simulink model "UpgradedConveyorBeltMechanism"  (R2023a)
settings: Solver=VariableStepAuto  StartTime=0.0  StopTime=30  RelTol=1e-3
values from neighbouring files (symbols this model uses):
  b = 40.6518    [UpgradedConveyorBeltParameters.m]
  B1 = 0.0042    [UpgradedConveyorBeltParameters.m]
  B2 = 0.0084    [UpgradedConveyorBeltParameters.m]
  J1 = 7e-5    (= 7e-05)    [UpgradedConveyorBeltParameters.m]
  J2 = 8e-5    (= 8e-05)    [UpgradedConveyorBeltParameters.m]
  k1 = 2.6552e5    (= 265520)    [UpgradedConveyorBeltParameters.m]
  k2 = 2.6552e5    (= 265520)    [UpgradedConveyorBeltParameters.m]
  k3 = 11.777e4    (= 117770)    [UpgradedConveyorBeltParameters.m]
  Kb = 23e-3    (= 0.023)    [UpgradedConveyorBeltParameters.m]
  Kt = 23e-3    (= 0.023)    [UpgradedConveyorBeltParameters.m]
  L = 0.1    [UpgradedConveyorBeltParameters.m]
  m = 2    [UpgradedConveyorBeltParameters.m]
  R = 0.71    [UpgradedConveyorBeltParameters.m]
  r = 0.0194    [UpgradedConveyorBeltParameters.m]
undefined symbols (not defined in the file or in its folder): J, Kd, Ke
libraries: fl_lib x20, slpidlib x10, fl_ps_legacy_lib x8, nesl_utility x6, SignalEditorBlockLib x5, ee_lib x2, simulink x1
(part 2 of 2)

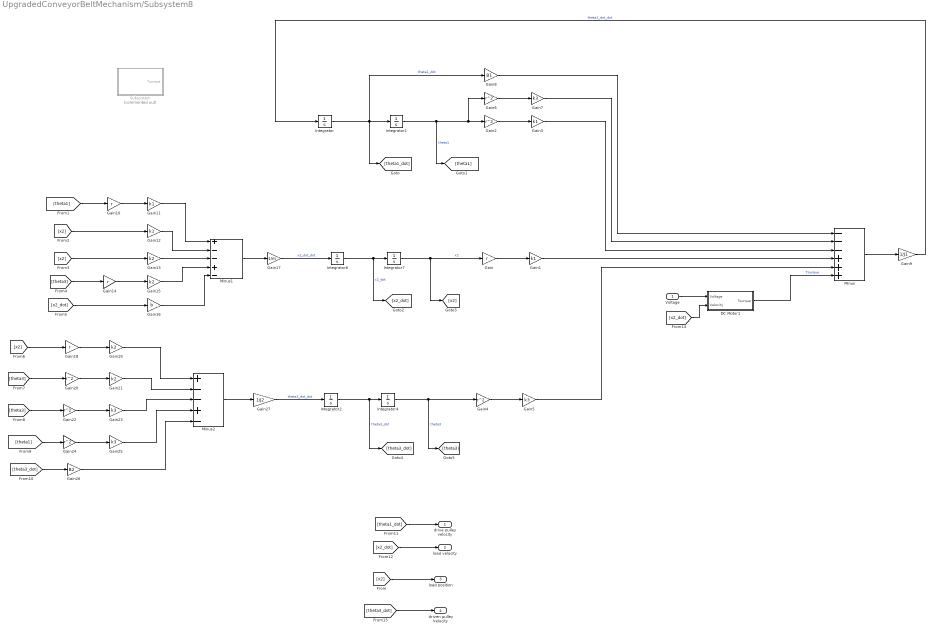
== system UpgradedConveyorBeltMechanism/Subsystem8 ==
  Voltage : Inport
  DC Motor1 : Subsystem
  Gain{,10,14,18} (4 alike) : Gain  Gain=r
  Gain{1,3,11..12} (4 alike) : Gain  Gain=k1
  Gain{13,15,19,21} (4 alike) : Gain  Gain=k2
  Gain16 : Gain  Gain=b
  Gain17 : Gain  Gain=1/m
  Gain{2,4,6,20,22,24} (6 alike) : Gain  Gain=r^2
  Gain{5,7,23,25} (4 alike) : Gain  Gain=k3
  Gain26 : Gain  Gain=B2
  Gain27 : Gain  Gain=1/J2
  Gain8 : Gain  Gain=B1
  Gain9 : Gain  Gain=1/J1
  Integrator{,1..2,4,6..7} (6 alike) : Integrator
  Minus : Sum  Inputs=---+++
  Minus1 : Sum  Inputs=+--+-
  Minus2 : Sum  Inputs=+--+-
  Subsystem : Subsystem  Commented=on
  drive pulley velocity : Outport
  load velocity : Outport  Port=2
  load position : Outport  Port=3
  driven pulley Velocity : Outport  Port=4
  wires:
  Gain23/1 -> Minus2/3
  Gain4/1 -> Gain5/1
  [theta1] -> Gain24/1
  Gain11/1 -> Minus1/1
  [theta3_dot] -> Gain26/1
  Gain26/1 -> Minus2/5
  Gain22/1 -> Gain23/1
  Gain19/1 -> Minus2/1
  Gain21/1 -> Minus2/2
  Integrator/1 -> Integrator1/1, [theta1_dot], Gain8/1  "theta1_dot"
  Integrator1/1 -> Gain6/1, Gain2/1, [theta1]  "theta1"
  Integrator6/1 -> Integrator7/1, [x2_dot]  "x2_dot"
  Gain3/1 -> Minus/3
  Gain18/1 -> Gain19/1
  Gain1/1 -> Minus/4
  Gain2/1 -> Gain3/1
  Integrator2/1 -> [theta3_dot], Integrator4/1  "theta3_dot"
  Integrator4/1 -> Gain4/1, [theta3]  "theta3"
  [x2] -> Gain12/1
  Gain/1 -> Gain1/1
  Gain10/1 -> Gain11/1
  Gain24/1 -> Gain25/1
  Gain13/1 -> Minus1/3
  [theta3] -> Gain20/1
  [theta3] -> Gain14/1
  Gain15/1 -> Minus1/4
  Gain6/1 -> Gain7/1
  [theta3] -> Gain22/1
  Gain5/1 -> Minus/5
  [theta1] -> Gain10/1
  [x2] -> Gain18/1
  Minus2/1 -> Gain27/1
  Minus1/1 -> Gain17/1
  Minus/1 -> Gain9/1
  Gain7/1 -> Minus/2
  Integrator7/1 -> Gain/1, [x2]  "x2"
  Gain16/1 -> Minus1/5
  Gain8/1 -> Minus/1
  Gain17/1 -> Integrator6/1  "x2_dot_dot"
  Gain14/1 -> Gain15/1
  Gain20/1 -> Gain21/1
  Gain9/1 -> Integrator/1  "theta1_dot_dot"
  Gain12/1 -> Minus1/2
  Gain25/1 -> Minus2/4
  [x2] -> Gain13/1
  [x2_dot] -> Gain16/1
  [theta1_dot] -> drive pulley velocity/1
  [x2_dot] -> load velocity/1
  Gain27/1 -> Integrator2/1  "theta3_dot_dot"
  DC Motor1/1(Tourque) -> Minus/6  "Tourque"
  [x2_dot] -> DC Motor1/2(Velocity)
  Voltage/1 -> DC Motor1/1(Voltage)
  [x2] -> load position/1
  [theta3_dot] -> driven pulley Velocity/1

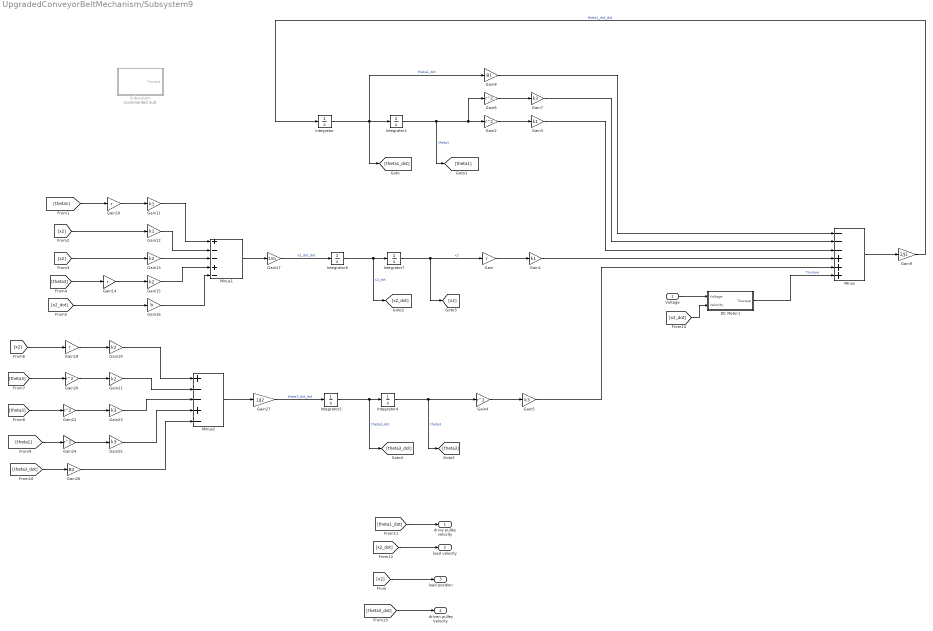
== system UpgradedConveyorBeltMechanism/Subsystem9 ==
  Voltage : Inport
  DC Motor1 : Subsystem
  Gain{,10,14,18} (4 alike) : Gain  Gain=r
  Gain{1,3,11..12} (4 alike) : Gain  Gain=k1
  Gain{13,15,19,21} (4 alike) : Gain  Gain=k2
  Gain16 : Gain  Gain=b
  Gain17 : Gain  Gain=1/m
  Gain{2,4,6,20,22,24} (6 alike) : Gain  Gain=r^2
  Gain{5,7,23,25} (4 alike) : Gain  Gain=k3
  Gain26 : Gain  Gain=B2
  Gain27 : Gain  Gain=1/J2
  Gain8 : Gain  Gain=B1
  Gain9 : Gain  Gain=1/J1
  Integrator{,1..2,4,6..7} (6 alike) : Integrator
  Minus : Sum  Inputs=---+++
  Minus1 : Sum  Inputs=+--+-
  Minus2 : Sum  Inputs=+--+-
  Subsystem : Subsystem  Commented=on
  drive pulley velocity : Outport
  load velocity : Outport  Port=2
  load position : Outport  Port=3
  driven pulley Velocity : Outport  Port=4
  wires:
  Gain23/1 -> Minus2/3
  Gain4/1 -> Gain5/1
  [theta1] -> Gain24/1
  Gain11/1 -> Minus1/1
  [theta3_dot] -> Gain26/1
  Gain26/1 -> Minus2/5
  Gain22/1 -> Gain23/1
  Gain19/1 -> Minus2/1
  Gain21/1 -> Minus2/2
  Integrator/1 -> Integrator1/1, [theta1_dot], Gain8/1  "theta1_dot"
  Integrator1/1 -> Gain6/1, Gain2/1, [theta1]  "theta1"
  Integrator6/1 -> Integrator7/1, [x2_dot]  "x2_dot"
  Gain3/1 -> Minus/3
  Gain18/1 -> Gain19/1
  Gain1/1 -> Minus/4
  Gain2/1 -> Gain3/1
  Integrator2/1 -> [theta3_dot], Integrator4/1  "theta3_dot"
  Integrator4/1 -> Gain4/1, [theta3]  "theta3"
  [x2] -> Gain12/1
  Gain/1 -> Gain1/1
  Gain10/1 -> Gain11/1
  Gain24/1 -> Gain25/1
  Gain13/1 -> Minus1/3
  [theta3] -> Gain20/1
  [theta3] -> Gain14/1
  Gain15/1 -> Minus1/4
  Gain6/1 -> Gain7/1
  [theta3] -> Gain22/1
  Gain5/1 -> Minus/5
  [theta1] -> Gain10/1
  [x2] -> Gain18/1
  Minus2/1 -> Gain27/1
  Minus1/1 -> Gain17/1
  Minus/1 -> Gain9/1
  Gain7/1 -> Minus/2
  Integrator7/1 -> Gain/1, [x2]  "x2"
  Gain16/1 -> Minus1/5
  Gain8/1 -> Minus/1
  Gain17/1 -> Integrator6/1  "x2_dot_dot"
  Gain14/1 -> Gain15/1
  Gain20/1 -> Gain21/1
  Gain9/1 -> Integrator/1  "theta1_dot_dot"
  Gain12/1 -> Minus1/2
  Gain25/1 -> Minus2/4
  [x2] -> Gain13/1
  [x2_dot] -> Gain16/1
  [theta1_dot] -> drive pulley velocity/1
  [x2_dot] -> load velocity/1
  Gain27/1 -> Integrator2/1  "theta3_dot_dot"
  DC Motor1/1(Tourque) -> Minus/6  "Tourque"
  [x2_dot] -> DC Motor1/2(Velocity)
  Voltage/1 -> DC Motor1/1(Voltage)
  [x2] -> load position/1
  [theta3_dot] -> driven pulley Velocity/1

== system UpgradedConveyorBeltMechanism/Controller/Position ==
  Ref : Inport
  Algorithm and Pulse Generation : Subsystem
  ERef : fl_lib/Electrical/Electrical Elements/Electrical Reference
  PWM : PMIOPort  Side=Right
  0v : PMIOPort  Port=2  Side=Right
  REV : PMIOPort  Port=3  Side=Right
  wires:
  Ref/1 -> Algorithm and Pulse Generation/1(Reference)
  connections:
  Algorithm and Pulse Generation/RConn2 -- PWM/RConn1
  Algorithm and Pulse Generation/RConn1 -- REV/RConn1
  ERef/LConn1 -- 0v/RConn1

== system UpgradedConveyorBeltMechanism/Controller/Speed ==
  note: Step rate and direction algorithm implemented on a microprocessor or dedicated discrete chip
  Ref : Inport
  ERef : fl_lib/Electrical/Electrical Elements/Electrical Reference
  Step Rate and Direction : Subsystem
  Voltage-Controlled Pulse Generator : Subsystem
  PWM : PMIOPort  Side=Right
  0v : PMIOPort  Port=2  Side=Right
  REV : PMIOPort  Port=3  Side=Right
  wires:
  Ref/1 -> Step Rate and Direction/1(Reference)
  connections:
  PWM/RConn1 -- Voltage-Controlled Pulse Generator/RConn1
  Voltage-Controlled Pulse Generator/RConn2 -- 0v/RConn1 -- ERef/LConn1
  Step Rate and Direction/RConn1 -- REV/RConn1
  Step Rate and Direction/RConn2 -- Voltage-Controlled Pulse Generator/LConn1

== system UpgradedConveyorBeltMechanism/Subsystem/DC Motor1 ==
  note: Armature Controlled DC Motor
      |
      | $E_a = R_a \cdot I_a + L_a \cdot \frac{di_a}{dt} + K_b \cdot \frac{d\theta}{dt}$
      | $T_{m} = K_{t} \cdot I_{a}$
  Voltage : Inport
  Velocity : Inport  Port=2
  Constant1 : Constant  Value=R
  Gain1 : Gain  Gain=Kb
  Gain2 : Gain  Gain=1/L
  Gain3 : Gain  Gain=Kt
  Integrator : Integrator
  Product : Product
  Subtract : Sum  Inputs=+--
  Tourque : Outport
  wires:
  Voltage/1 -> Subtract/1
  Integrator/1 -> Product/1, Gain3/1  "i"
  Gain3/1 -> Tourque/1
  Gain1/1 -> Subtract/2
  Velocity/1 -> Gain1/1
  Constant1/1 -> Product/2
  Product/1 -> Subtract/3
  Gain2/1 -> Integrator/1  "i_dot"
  Subtract/1 -> Gain2/1

== system UpgradedConveyorBeltMechanism/Subsystem1/DC Motor1 ==
  note: Armature Controlled DC Motor
      |
      | $E_a = R_a \cdot I_a + L_a \cdot \frac{di_a}{dt} + K_b \cdot \frac{d\theta}{dt}$
      | $T_{m} = K_{t} \cdot I_{a}$
  Voltage : Inport
  Velocity : Inport  Port=2
  Constant1 : Constant  Value=R
  Gain1 : Gain  Gain=Kb
  Gain2 : Gain  Gain=1/L
  Gain3 : Gain  Gain=Kt
  Integrator : Integrator
  Product : Product
  Subtract : Sum  Inputs=+--
  Tourque : Outport
  wires:
  Voltage/1 -> Subtract/1
  Integrator/1 -> Product/1, Gain3/1  "i"
  Gain3/1 -> Tourque/1
  Gain1/1 -> Subtract/2
  Velocity/1 -> Gain1/1
  Constant1/1 -> Product/2
  Product/1 -> Subtract/3
  Gain2/1 -> Integrator/1  "i_dot"
  Subtract/1 -> Gain2/1

== system UpgradedConveyorBeltMechanism/Subsystem1/Subsystem ==
  Constant : Constant  Value=Kt
  Constant1 : Constant  Value=Ke
  Constant2 : Constant  Value=R
  Divide : Product  Inputs=**/
  Divide1 : Product  Inputs=***/
  Minus3 : Sum  Inputs=+-
  Voltage : DiscretePulseGenerator  PulseType=Time based  Amplitude=12  Period=11  PulseWidth=50  PhaseDelay=2
  Tourque : Outport
  wires:
  Divide1/1 -> Minus3/2
  Divide/1 -> Minus3/1
  Constant/1 -> Divide/2, Divide1/1
  [theta1_dot] -> Divide1/3
  Constant1/1 -> Divide1/2
  Constant2/1 -> Divide1/4, Divide/3
  Minus3/1 -> Tourque/1  "Tourque"
  Voltage/1 -> Divide/1

== system UpgradedConveyorBeltMechanism/Subsystem10/DC Motor1 ==
  note: Armature Controlled DC Motor
      |
      | $E_a = R_a \cdot I_a + L_a \cdot \frac{di_a}{dt} + K_b \cdot \frac{d\theta}{dt}$
      | $T_{m} = K_{t} \cdot I_{a}$
  Voltage : Inport
  Velocity : Inport  Port=2
  Constant1 : Constant  Value=R
  Gain1 : Gain  Gain=Kb
  Gain2 : Gain  Gain=1/L
  Gain3 : Gain  Gain=Kt
  Integrator : Integrator
  Product : Product
  Subtract : Sum  Inputs=+--
  Tourque : Outport
  wires:
  Voltage/1 -> Subtract/1
  Integrator/1 -> Product/1, Gain3/1  "i"
  Gain3/1 -> Tourque/1
  Gain1/1 -> Subtract/2
  Velocity/1 -> Gain1/1
  Constant1/1 -> Product/2
  Product/1 -> Subtract/3
  Gain2/1 -> Integrator/1  "i_dot"
  Subtract/1 -> Gain2/1

== system UpgradedConveyorBeltMechanism/Subsystem10/Subsystem ==
  Constant : Constant  Value=Kt
  Constant1 : Constant  Value=Ke
  Constant2 : Constant  Value=R
  Divide : Product  Inputs=**/
  Divide1 : Product  Inputs=***/
  Minus3 : Sum  Inputs=+-
  Voltage : DiscretePulseGenerator  PulseType=Time based  Amplitude=12  Period=11  PulseWidth=50  PhaseDelay=2
  Tourque : Outport
  wires:
  Divide1/1 -> Minus3/2
  Divide/1 -> Minus3/1
  Constant/1 -> Divide/2, Divide1/1
  [theta1_dot] -> Divide1/3
  Constant1/1 -> Divide1/2
  Constant2/1 -> Divide1/4, Divide/3
  Minus3/1 -> Tourque/1  "Tourque"
  Voltage/1 -> Divide/1

== system UpgradedConveyorBeltMechanism/Subsystem2/DC Motor1 ==
  note: Armature Controlled DC Motor
      |
      | $E_a = R_a \cdot I_a + L_a \cdot \frac{di_a}{dt} + K_b \cdot \frac{d\theta}{dt}$
      | $T_{m} = K_{t} \cdot I_{a}$
  Voltage : Inport
  Velocity : Inport  Port=2
  Constant1 : Constant  Value=R
  Gain1 : Gain  Gain=Kb
  Gain2 : Gain  Gain=1/L
  Gain3 : Gain  Gain=Kt
  Integrator : Integrator
  Product : Product
  Subtract : Sum  Inputs=+--
  Tourque : Outport
  wires:
  Voltage/1 -> Subtract/1
  Integrator/1 -> Product/1, Gain3/1  "i"
  Gain3/1 -> Tourque/1
  Gain1/1 -> Subtract/2
  Velocity/1 -> Gain1/1
  Constant1/1 -> Product/2
  Product/1 -> Subtract/3
  Gain2/1 -> Integrator/1  "i_dot"
  Subtract/1 -> Gain2/1

== system UpgradedConveyorBeltMechanism/Subsystem2/Subsystem ==
  Constant : Constant  Value=Kt
  Constant1 : Constant  Value=Ke
  Constant2 : Constant  Value=R
  Divide : Product  Inputs=**/
  Divide1 : Product  Inputs=***/
  Minus3 : Sum  Inputs=+-
  Voltage : DiscretePulseGenerator  PulseType=Time based  Amplitude=12  Period=11  PulseWidth=50  PhaseDelay=2
  Tourque : Outport
  wires:
  Divide1/1 -> Minus3/2
  Divide/1 -> Minus3/1
  Constant/1 -> Divide/2, Divide1/1
  [theta1_dot] -> Divide1/3
  Constant1/1 -> Divide1/2
  Constant2/1 -> Divide1/4, Divide/3
  Minus3/1 -> Tourque/1  "Tourque"
  Voltage/1 -> Divide/1

== system UpgradedConveyorBeltMechanism/Subsystem3/DC Motor1 ==
  note: Armature Controlled DC Motor
      |
      | $E_a = R_a \cdot I_a + L_a \cdot \frac{di_a}{dt} + K_b \cdot \frac{d\theta}{dt}$
      | $T_{m} = K_{t} \cdot I_{a}$
  Voltage : Inport
  Velocity : Inport  Port=2
  Constant1 : Constant  Value=R
  Gain1 : Gain  Gain=Kb
  Gain2 : Gain  Gain=1/L
  Gain3 : Gain  Gain=Kt
  Integrator : Integrator
  Product : Product
  Subtract : Sum  Inputs=+--
  Tourque : Outport
  wires:
  Voltage/1 -> Subtract/1
  Integrator/1 -> Product/1, Gain3/1  "i"
  Gain3/1 -> Tourque/1
  Gain1/1 -> Subtract/2
  Velocity/1 -> Gain1/1
  Constant1/1 -> Product/2
  Product/1 -> Subtract/3
  Gain2/1 -> Integrator/1  "i_dot"
  Subtract/1 -> Gain2/1

== system UpgradedConveyorBeltMechanism/Subsystem3/Subsystem ==
  Constant : Constant  Value=Kt
  Constant1 : Constant  Value=Ke
  Constant2 : Constant  Value=R
  Divide : Product  Inputs=**/
  Divide1 : Product  Inputs=***/
  Minus3 : Sum  Inputs=+-
  Voltage : DiscretePulseGenerator  PulseType=Time based  Amplitude=12  Period=11  PulseWidth=50  PhaseDelay=2
  Tourque : Outport
  wires:
  Divide1/1 -> Minus3/2
  Divide/1 -> Minus3/1
  Constant/1 -> Divide/2, Divide1/1
  [theta1_dot] -> Divide1/3
  Constant1/1 -> Divide1/2
  Constant2/1 -> Divide1/4, Divide/3
  Minus3/1 -> Tourque/1  "Tourque"
  Voltage/1 -> Divide/1

== system UpgradedConveyorBeltMechanism/Subsystem4/DC Motor1 ==
  note: Armature Controlled DC Motor
      |
      | $E_a = R_a \cdot I_a + L_a \cdot \frac{di_a}{dt} + K_b \cdot \frac{d\theta}{dt}$
      | $T_{m} = K_{t} \cdot I_{a}$
  Voltage : Inport
  Velocity : Inport  Port=2
  Constant1 : Constant  Value=R
  Gain1 : Gain  Gain=Kb
  Gain2 : Gain  Gain=1/L
  Gain3 : Gain  Gain=Kt
  Integrator : Integrator
  Product : Product
  Subtract : Sum  Inputs=+--
  Tourque : Outport
  wires:
  Voltage/1 -> Subtract/1
  Integrator/1 -> Product/1, Gain3/1  "i"
  Gain3/1 -> Tourque/1
  Gain1/1 -> Subtract/2
  Velocity/1 -> Gain1/1
  Constant1/1 -> Product/2
  Product/1 -> Subtract/3
  Gain2/1 -> Integrator/1  "i_dot"
  Subtract/1 -> Gain2/1

== system UpgradedConveyorBeltMechanism/Subsystem4/Subsystem ==
  Constant : Constant  Value=Kt
  Constant1 : Constant  Value=Ke
  Constant2 : Constant  Value=R
  Divide : Product  Inputs=**/
  Divide1 : Product  Inputs=***/
  Minus3 : Sum  Inputs=+-
  Voltage : DiscretePulseGenerator  PulseType=Time based  Amplitude=12  Period=11  PulseWidth=50  PhaseDelay=2
  Tourque : Outport
  wires:
  Divide1/1 -> Minus3/2
  Divide/1 -> Minus3/1
  Constant/1 -> Divide/2, Divide1/1
  [theta1_dot] -> Divide1/3
  Constant1/1 -> Divide1/2
  Constant2/1 -> Divide1/4, Divide/3
  Minus3/1 -> Tourque/1  "Tourque"
  Voltage/1 -> Divide/1

== system UpgradedConveyorBeltMechanism/Subsystem5/DC Motor1 ==
  note: Armature Controlled DC Motor
      |
      | $E_a = R_a \cdot I_a + L_a \cdot \frac{di_a}{dt} + K_b \cdot \frac{d\theta}{dt}$
      | $T_{m} = K_{t} \cdot I_{a}$
  Voltage : Inport
  Velocity : Inport  Port=2
  Constant1 : Constant  Value=R
  Gain1 : Gain  Gain=Kb
  Gain2 : Gain  Gain=1/L
  Gain3 : Gain  Gain=Kt
  Integrator : Integrator
  Product : Product
  Subtract : Sum  Inputs=+--
  Tourque : Outport
  wires:
  Voltage/1 -> Subtract/1
  Integrator/1 -> Product/1, Gain3/1  "i"
  Gain3/1 -> Tourque/1
  Gain1/1 -> Subtract/2
  Velocity/1 -> Gain1/1
  Constant1/1 -> Product/2
  Product/1 -> Subtract/3
  Gain2/1 -> Integrator/1  "i_dot"
  Subtract/1 -> Gain2/1

== system UpgradedConveyorBeltMechanism/Subsystem5/Subsystem ==
  Constant : Constant  Value=Kt
  Constant1 : Constant  Value=Ke
  Constant2 : Constant  Value=R
  Divide : Product  Inputs=**/
  Divide1 : Product  Inputs=***/
  Minus3 : Sum  Inputs=+-
  Voltage : DiscretePulseGenerator  PulseType=Time based  Amplitude=12  Period=11  PulseWidth=50  PhaseDelay=2
  Tourque : Outport
  wires:
  Divide1/1 -> Minus3/2
  Divide/1 -> Minus3/1
  Constant/1 -> Divide/2, Divide1/1
  [theta1_dot] -> Divide1/3
  Constant1/1 -> Divide1/2
  Constant2/1 -> Divide1/4, Divide/3
  Minus3/1 -> Tourque/1  "Tourque"
  Voltage/1 -> Divide/1

== system UpgradedConveyorBeltMechanism/Subsystem6/DC Motor1 ==
  note: Armature Controlled DC Motor
      |
      | $E_a = R_a \cdot I_a + L_a \cdot \frac{di_a}{dt} + K_b \cdot \frac{d\theta}{dt}$
      | $T_{m} = K_{t} \cdot I_{a}$
  Voltage : Inport
  Velocity : Inport  Port=2
  Constant1 : Constant  Value=R
  Gain1 : Gain  Gain=Kb
  Gain2 : Gain  Gain=1/L
  Gain3 : Gain  Gain=Kt
  Integrator : Integrator
  Product : Product
  Subtract : Sum  Inputs=+--
  Tourque : Outport
  wires:
  Voltage/1 -> Subtract/1
  Integrator/1 -> Product/1, Gain3/1  "i"
  Gain3/1 -> Tourque/1
  Gain1/1 -> Subtract/2
  Velocity/1 -> Gain1/1
  Constant1/1 -> Product/2
  Product/1 -> Subtract/3
  Gain2/1 -> Integrator/1  "i_dot"
  Subtract/1 -> Gain2/1

== system UpgradedConveyorBeltMechanism/Subsystem6/Subsystem ==
  Constant : Constant  Value=Kt
  Constant1 : Constant  Value=Ke
  Constant2 : Constant  Value=R
  Divide : Product  Inputs=**/
  Divide1 : Product  Inputs=***/
  Minus3 : Sum  Inputs=+-
  Voltage : DiscretePulseGenerator  PulseType=Time based  Amplitude=12  Period=11  PulseWidth=50  PhaseDelay=2
  Tourque : Outport
  wires:
  Divide1/1 -> Minus3/2
  Divide/1 -> Minus3/1
  Constant/1 -> Divide/2, Divide1/1
  [theta1_dot] -> Divide1/3
  Constant1/1 -> Divide1/2
  Constant2/1 -> Divide1/4, Divide/3
  Minus3/1 -> Tourque/1  "Tourque"
  Voltage/1 -> Divide/1

== system UpgradedConveyorBeltMechanism/Subsystem7/DC Motor1 ==
  note: Armature Controlled DC Motor
      |
      | $E_a = R_a \cdot I_a + L_a \cdot \frac{di_a}{dt} + K_b \cdot \frac{d\theta}{dt}$
      | $T_{m} = K_{t} \cdot I_{a}$
  Voltage : Inport
  Velocity : Inport  Port=2
  Constant1 : Constant  Value=R
  Gain1 : Gain  Gain=Kb
  Gain2 : Gain  Gain=1/L
  Gain3 : Gain  Gain=Kt
  Integrator : Integrator
  Product : Product
  Subtract : Sum  Inputs=+--
  Tourque : Outport
  wires:
  Voltage/1 -> Subtract/1
  Integrator/1 -> Product/1, Gain3/1  "i"
  Gain3/1 -> Tourque/1
  Gain1/1 -> Subtract/2
  Velocity/1 -> Gain1/1
  Constant1/1 -> Product/2
  Product/1 -> Subtract/3
  Gain2/1 -> Integrator/1  "i_dot"
  Subtract/1 -> Gain2/1

== system UpgradedConveyorBeltMechanism/Subsystem7/Subsystem ==
  Constant : Constant  Value=Kt
  Constant1 : Constant  Value=Ke
  Constant2 : Constant  Value=R
  Divide : Product  Inputs=**/
  Divide1 : Product  Inputs=***/
  Minus3 : Sum  Inputs=+-
  Voltage : DiscretePulseGenerator  PulseType=Time based  Amplitude=12  Period=11  PulseWidth=50  PhaseDelay=2
  Tourque : Outport
  wires:
  Divide1/1 -> Minus3/2
  Divide/1 -> Minus3/1
  Constant/1 -> Divide/2, Divide1/1
  [theta1_dot] -> Divide1/3
  Constant1/1 -> Divide1/2
  Constant2/1 -> Divide1/4, Divide/3
  Minus3/1 -> Tourque/1  "Tourque"
  Voltage/1 -> Divide/1

== system UpgradedConveyorBeltMechanism/Subsystem8/DC Motor1 ==
  note: Armature Controlled DC Motor
      |
      | $E_a = R_a \cdot I_a + L_a \cdot \frac{di_a}{dt} + K_b \cdot \frac{d\theta}{dt}$
      | $T_{m} = K_{t} \cdot I_{a}$
  Voltage : Inport
  Velocity : Inport  Port=2
  Constant1 : Constant  Value=R
  Gain1 : Gain  Gain=Kb
  Gain2 : Gain  Gain=1/L
  Gain3 : Gain  Gain=Kt
  Integrator : Integrator
  Product : Product
  Subtract : Sum  Inputs=+--
  Tourque : Outport
  wires:
  Voltage/1 -> Subtract/1
  Integrator/1 -> Product/1, Gain3/1  "i"
  Gain3/1 -> Tourque/1
  Gain1/1 -> Subtract/2
  Velocity/1 -> Gain1/1
  Constant1/1 -> Product/2
  Product/1 -> Subtract/3
  Gain2/1 -> Integrator/1  "i_dot"
  Subtract/1 -> Gain2/1

== system UpgradedConveyorBeltMechanism/Subsystem8/Subsystem ==
  Constant : Constant  Value=Kt
  Constant1 : Constant  Value=Ke
  Constant2 : Constant  Value=R
  Divide : Product  Inputs=**/
  Divide1 : Product  Inputs=***/
  Minus3 : Sum  Inputs=+-
  Voltage : DiscretePulseGenerator  PulseType=Time based  Amplitude=12  Period=11  PulseWidth=50  PhaseDelay=2
  Tourque : Outport
  wires:
  Divide1/1 -> Minus3/2
  Divide/1 -> Minus3/1
  Constant/1 -> Divide/2, Divide1/1
  [theta1_dot] -> Divide1/3
  Constant1/1 -> Divide1/2
  Constant2/1 -> Divide1/4, Divide/3
  Minus3/1 -> Tourque/1  "Tourque"
  Voltage/1 -> Divide/1

== system UpgradedConveyorBeltMechanism/Subsystem9/DC Motor1 ==
  note: Armature Controlled DC Motor
      |
      | $E_a = R_a \cdot I_a + L_a \cdot \frac{di_a}{dt} + K_b \cdot \frac{d\theta}{dt}$
      | $T_{m} = K_{t} \cdot I_{a}$
  Voltage : Inport
  Velocity : Inport  Port=2
  Constant1 : Constant  Value=R
  Gain1 : Gain  Gain=Kb
  Gain2 : Gain  Gain=1/L
  Gain3 : Gain  Gain=Kt
  Integrator : Integrator
  Product : Product
  Subtract : Sum  Inputs=+--
  Tourque : Outport
  wires:
  Voltage/1 -> Subtract/1
  Integrator/1 -> Product/1, Gain3/1  "i"
  Gain3/1 -> Tourque/1
  Gain1/1 -> Subtract/2
  Velocity/1 -> Gain1/1
  Constant1/1 -> Product/2
  Product/1 -> Subtract/3
  Gain2/1 -> Integrator/1  "i_dot"
  Subtract/1 -> Gain2/1

== system UpgradedConveyorBeltMechanism/Subsystem9/Subsystem ==
  Constant : Constant  Value=Kt
  Constant1 : Constant  Value=Ke
  Constant2 : Constant  Value=R
  Divide : Product  Inputs=**/
  Divide1 : Product  Inputs=***/
  Minus3 : Sum  Inputs=+-
  Voltage : DiscretePulseGenerator  PulseType=Time based  Amplitude=12  Period=11  PulseWidth=50  PhaseDelay=2
  Tourque : Outport
  wires:
  Divide1/1 -> Minus3/2
  Divide/1 -> Minus3/1
  Constant/1 -> Divide/2, Divide1/1
  [theta1_dot] -> Divide1/3
  Constant1/1 -> Divide1/2
  Constant2/1 -> Divide1/4, Divide/3
  Minus3/1 -> Tourque/1  "Tourque"
  Voltage/1 -> Divide/1

== system UpgradedConveyorBeltMechanism/Controller/Position/Algorithm and Pulse Generation ==
  note: The reference input defines the required angular position in terms of
      | the number steps. For this stepper, the step size is 1.8 degrees. Hence
      | a demand of 10 steps results in an angle change of 18 degrees.
      | The step rate is set by the Pulse Generator's Pulse rate mask parameter.
  note: Position Controller
  Reference : Inport
  IC Analog Output REV : Subsystem
  IC Analog Output Vref : Subsystem
  Logic2Volts1 : Gain  Gain=5
  Logic2Volts2 : Gain  Gain=5
  Pulse Generator : Subsystem  mask{f=20}
      mask prompts: f "Pulse rate"
  Rate Transition : RateTransition  Deterministic=off
  REV : PMIOPort  Side=Right
  Vref : PMIOPort  Port=2  Side=Right
  wires:
  Logic2Volts1/1 -> IC Analog Output Vref/1(SL)
  Pulse Generator/1(Pulse train) -> Logic2Volts1/1
  Reference/1 -> Rate Transition/1
  Logic2Volts2/1 -> IC Analog Output REV/1(SL)
  Pulse Generator/2(Pulse direction) -> Logic2Volts2/1
  Rate Transition/1 -> Pulse Generator/1(Pulse  demand)
  connections:
  Vref/RConn1 -- IC Analog Output Vref/RConn1
  REV/RConn1 -- IC Analog Output REV/RConn1

== system UpgradedConveyorBeltMechanism/Controller/Speed/Step Rate and Direction ==
  note: The speed controller turns the reference input into an absolute voltage demand for the
      | voltage-controlled pulse generator and sets the reverse flag signal to +5 volts when the
      | speed demand is negative.
  Reference : Inport
  Abs : Abs  SaturateOnIntegerOverflow=off
  Compare To Constant : simulink/Logic and Bit Operations/Compare To Constant  relop=<  const=0  OutDataTypeStr=uint8  ZeroCross=off
  Data Type Conversion : DataTypeConversion  SaturateOnIntegerOverflow=off  RndMeth=Floor
  IC Analog Output REV : Subsystem
  IC Analog Output Vref : Subsystem
  Logic2Volts : Gain  Gain=5
  Max step rate 100/s : Saturate  UpperLimit=100  LowerLimit=0
  StepRate2Volts : Gain  Gain=5/100
  REV : PMIOPort  Side=Right
  Vref : PMIOPort  Port=2  Side=Right
  wires:
  StepRate2Volts/1 -> IC Analog Output Vref/1(SL)
  Max step rate 100/s/1 -> StepRate2Volts/1
  Data Type Conversion/1 -> Logic2Volts/1
  Compare To Constant/1 -> Data Type Conversion/1
  Reference/1 -> Compare To Constant/1, Abs/1
  Abs/1 -> Max step rate 100/s/1
  Logic2Volts/1 -> IC Analog Output REV/1(SL)
  connections:
  REV/RConn1 -- IC Analog Output REV/RConn1
  Vref/RConn1 -- IC Analog Output Vref/RConn1

== system UpgradedConveyorBeltMechanism/Controller/Speed/Voltage-Controlled Pulse Generator ==
  2*pi : fl_ps_legacy_lib/Legacy Physical Signals/Functions/PS Gain  gain=-2*pi
  Controlled Voltage Source : fl_lib/Electrical/Electrical Sources/Controlled Voltage Source
  ERef : fl_lib/Electrical/Electrical Elements/Electrical Reference
  Max step rate =100 : fl_ps_legacy_lib/Legacy Physical Signals/Functions/PS Gain  gain=100
  Normalize to 1 : fl_ps_legacy_lib/Legacy Physical Signals/Functions/PS Gain  gain=1/5
  PS Integrator : fl_ps_legacy_lib/Legacy Physical Signals/Linear Operators/PS Integrator  x0=0
      settings: InternalSimscapePortConfiguration="{\"Bottom\":[],\"Left\":[{\"id\":\"I\",\"label\":\"\",\"type\":\"input\"}],\"Right\":[{\"id\":\"O\",\"label\":\"\",\"type\":\"output\"}],\"Top\":[]}"
  PS Sign : fl_ps_legacy_lib/Legacy Physical Signals/Nonlinear Operators/PS Sign
      settings: InternalSimscapePortConfiguration="{\"Bottom\":[],\"Left\":[{\"id\":\"I\",\"label\":\"\",\"type\":\"input\"}],\"Right\":[{\"id\":\"O\",\"label\":\"\",\"type\":\"output\"}],\"Top\":[]}"
  PS Sine : fl_ps_legacy_lib/Legacy Physical Signals/Functions/PS Math Function  fcn_choice=1
      settings: InternalSimscapePortConfiguration="{\"Bottom\":[],\"Left\":[{\"id\":\"I\",\"label\":\"\",\"type\":\"input\"}],\"Right\":[{\"id\":\"O\",\"label\":\"\",\"type\":\"output\"}],\"Top\":[]}"
  Voltage Sensor : fl_lib/Electrical/Electrical Sensors/Voltage Sensor
  "[0,1]" : fl_ps_legacy_lib/Legacy Physical Signals/Nonlinear Operators/PS Saturation  upper_limit=1  lower_limit=0
      settings: InternalSimscapePortConfiguration="{\"Bottom\":[],\"Left\":[{\"id\":\"I\",\"label\":\"\",\"type\":\"input\"}],\"Right\":[{\"id\":\"O\",\"label\":\"\",\"type\":\"output\"}],\"Top\":[]}"
  logic2volts : fl_ps_legacy_lib/Legacy Physical Signals/Functions/PS Gain  gain=5
  PWM : PMIOPort  Side=Right
  0v : PMIOPort  Port=2  Side=Right
  Vref : PMIOPort  Port=3  Side=Left
  connections:
  PWM/RConn1 -- Controlled Voltage Source/LConn1
  Controlled Voltage Source/RConn2 -- 0v/RConn1
  Vref/RConn1 -- Voltage Sensor/LConn1
  ERef/LConn1 -- Voltage Sensor/RConn2
  Voltage Sensor/RConn1 -- Normalize to 1/LConn1
  Max step rate =100/LConn1 -- Normalize to 1/RConn1
  Max step rate =100/RConn1 -- 2*pi/LConn1
  2*pi/RConn1 -- PS Integrator/LConn1
  PS Integrator/RConn1 -- PS Sine/LConn1
  PS Sign/LConn1 -- PS Sine/RConn1
  "[0,1]"/LConn1 -- PS Sign/RConn1
  "[0,1]"/RConn1 -- logic2volts/LConn1
  logic2volts/RConn1 -- Controlled Voltage Source/RConn1

== system UpgradedConveyorBeltMechanism/Controller/Position/Algorithm and Pulse Generation/IC Analog Output REV ==
  SL : Inport
  Controlled Voltage Source : fl_lib/Electrical/Electrical Sources/Controlled Voltage Source
  ERef : fl_lib/Electrical/Electrical Elements/Electrical Reference
  Simulink-PS Converter : nesl_utility/Simulink-PS Converter  PhysicalDomain=network_engine_domain  SubClassName=ps_input  LeftPortType=input  RightPortType=output  PseudoPeriodic=off  Frequencies=[]  NoiseDistribution=none  NoiseParameters=[]  Unit=V  AffineConversion=off  FilteringAndDerivatives=zero  SimscapeFilterOrder=1  InputFilterTimeConstant=.001  UdotUserProvided=0
  V : PMIOPort  Side=Right
  wires:
  SL/1 -> Simulink-PS Converter/1
  connections:
  ERef/LConn1 -- Controlled Voltage Source/RConn2
  V/RConn1 -- Controlled Voltage Source/LConn1
  Simulink-PS Converter/RConn1 -- Controlled Voltage Source/RConn1

== system UpgradedConveyorBeltMechanism/Controller/Position/Algorithm and Pulse Generation/IC Analog Output Vref ==
  SL : Inport
  Controlled Voltage Source : fl_lib/Electrical/Electrical Sources/Controlled Voltage Source
  ERef : fl_lib/Electrical/Electrical Elements/Electrical Reference
  Simulink-PS Converter : nesl_utility/Simulink-PS Converter  PhysicalDomain=network_engine_domain  SubClassName=ps_input  LeftPortType=input  RightPortType=output  PseudoPeriodic=off  Frequencies=[]  NoiseDistribution=none  NoiseParameters=[]  Unit=V  AffineConversion=off  FilteringAndDerivatives=zero  SimscapeFilterOrder=1  InputFilterTimeConstant=.001  UdotUserProvided=0
  V : PMIOPort  Side=Right
  wires:
  SL/1 -> Simulink-PS Converter/1
  connections:
  Simulink-PS Converter/RConn1 -- Controlled Voltage Source/RConn1
  V/RConn1 -- Controlled Voltage Source/LConn1
  ERef/LConn1 -- Controlled Voltage Source/RConn2

== system UpgradedConveyorBeltMechanism/Controller/Position/Algorithm and Pulse Generation/Pulse Generator ==
  Pulse  demand : Inport  SampleTime=1/f
  -1 : Gain  Gain=-1
  Abs : Abs  SaturateOnIntegerOverflow=off
  Product : Product  InputSameDT=on  SaturateOnIntegerOverflow=on  OutDataTypeStr=Inherit: Same as first input
  Pulse Generator : Subsystem
  Rate Transition : RateTransition  Deterministic=off
  Saturation : Saturate  UpperLimit=1  LowerLimit=-1
  Sign : Signum
  Sum : Sum  Inputs=|+-
  Sum1 : Sum  Inputs=|++
  "Unit Delay, sample time 1/f" : UnitDelay  SampleTime=1/f  HasFrameUpgradeWarning=on
  "[0,1]" : Saturate  UpperLimit=1  LowerLimit=0
  Pulse train : Outport  VectorParamsAs1DForOutWhenUnconnected=off
  Pulse direction : Outport  Port=2  VectorParamsAs1DForOutWhenUnconnected=off
  wires:
  "[0,1]"/1 -> Pulse direction/1
  -1/1 -> Sign/1
  "Unit Delay, sample time 1/f"/1 -> Sum/2, Sum1/2
  Pulse  demand/1 -> Sum/1
  Sum/1 -> -1/1, Saturation/1
  Saturation/1 -> Sum1/1, Abs/1
  Sum1/1 -> "Unit Delay, sample time 1/f"/1
  Sign/1 -> "[0,1]"/1
  Product/1 -> Pulse train/1
  Abs/1 -> Rate Transition/1
  Pulse Generator/1(p) -> Product/2
  Rate Transition/1 -> Product/1

== system UpgradedConveyorBeltMechanism/Controller/Speed/Step Rate and Direction/IC Analog Output REV ==
  SL : Inport
  Controlled Voltage Source : fl_lib/Electrical/Electrical Sources/Controlled Voltage Source
  ERef : fl_lib/Electrical/Electrical Elements/Electrical Reference
  Simulink-PS Converter : nesl_utility/Simulink-PS Converter  PhysicalDomain=network_engine_domain  SubClassName=ps_input  LeftPortType=input  RightPortType=output  PseudoPeriodic=off  Frequencies=[]  NoiseDistribution=none  NoiseParameters=[]  Unit=V  AffineConversion=off  FilteringAndDerivatives=zero  SimscapeFilterOrder=1  InputFilterTimeConstant=.001  UdotUserProvided=0
  V : PMIOPort  Side=Right
  wires:
  SL/1 -> Simulink-PS Converter/1
  connections:
  Simulink-PS Converter/RConn1 -- Controlled Voltage Source/RConn1
  V/RConn1 -- Controlled Voltage Source/LConn1
  ERef/LConn1 -- Controlled Voltage Source/RConn2

== system UpgradedConveyorBeltMechanism/Controller/Speed/Step Rate and Direction/IC Analog Output Vref ==
  SL : Inport
  Controlled Voltage Source : fl_lib/Electrical/Electrical Sources/Controlled Voltage Source
  ERef : fl_lib/Electrical/Electrical Elements/Electrical Reference
  Simulink-PS Converter : nesl_utility/Simulink-PS Converter  PhysicalDomain=network_engine_domain  SubClassName=ps_input  LeftPortType=input  RightPortType=output  PseudoPeriodic=off  Frequencies=[]  NoiseDistribution=none  NoiseParameters=[]  Unit=V  AffineConversion=off  FilteringAndDerivatives=zero  SimscapeFilterOrder=1  InputFilterTimeConstant=.001  UdotUserProvided=0
  V : PMIOPort  Side=Right
  wires:
  SL/1 -> Simulink-PS Converter/1
  connections:
  ERef/LConn1 -- Controlled Voltage Source/RConn2
  V/RConn1 -- Controlled Voltage Source/LConn1
  Simulink-PS Converter/RConn1 -- Controlled Voltage Source/RConn1

== system UpgradedConveyorBeltMechanism/Controller/Position/Algorithm and Pulse Generation/Pulse Generator/Pulse Generator ==
  -1 : Gain  Gain=0.5
  Constant : Constant  SampleTime=1/(2*f)
  Gain : Gain  Gain=-1
  Sum : Sum  Inputs=|++
  "Unit Delay, sample time 1/2*f)" : UnitDelay  InitialCondition=-1  SampleTime=1/(2*f)  HasFrameUpgradeWarning=on
  p : Outport  VectorParamsAs1DForOutWhenUnconnected=off
  wires:
  "Unit Delay, sample time 1/2*f)"/1 -> Gain/1, Sum/1
  Gain/1 -> "Unit Delay, sample time 1/2*f)"/1
  Constant/1 -> Sum/2
  Sum/1 -> -1/1
  -1/1 -> p/1

== matlab function UpgradedConveyorBeltMechanism/MATLAB Function ==
  data: x output; meal input; y output
function [x, y] = mealSelector(meal)
    % Initialize variables
    x = 0;
    y = 0;

    % Check the chosen meal
    switch meal
        case 1
            x = 1;
            y = 1;
        case 2
            x = 2;
            y = 2;
        case 3
            x = 3;
            y = 3;
        case 4
            x = 4;
            y = 4;
        case 5
            x = 5;
            y = 5;
        case 6
            x = 6;
            y = 6;
        case 7
            x = 7;
            y = 7;
        case 8
            x = 8;
            y = 8;
        case 9
            x = 9;
            y = 9;
        otherwise
            disp('Invalid option. No change to x and y.');
    end
end

== stateflow chart UpgradedConveyorBeltMechanism/Sensors ==
  state Stationery
    entry:
    Voltage=0;
  state Motion
    entry:
    Voltage=1;
  (default) -> Stationery
  Stationery -> Motion : [Crane==1]
  Motion -> Stationery : [Belt==1]
  data: Crane input; Belt input; Voltage output

== stateflow chart UpgradedConveyorBeltMechanism/Sensors Logic ==
  state Motor9
    entry:
    V9=12;
  state Motor8
    entry:
    V8=12;
  state Motor7
    entry:
    V7=12;
  state Motor1
    entry:
    V1=1;
  state Stationery
    entry:
    V1=0; V2=0; V3=0; V4=0; V5=0; V6=0;
    V7=0; V8=0; V9=0;
  state Motor2
    entry:
    V2=1;
  state Motor6
    entry:
    V6=12;
  state Motor3
    entry:
    V3=1;
  state Motor5
    entry:
    V5=12;
  state Motor4
    entry:
    V4=1;
  Stationery -> Motor8 [order 8] : [x==8&&y==8]
  Motor8 -> Stationery : [Belt8==1]
  Stationery -> Motor9 [order 9] : [x==9&&y==9]
  Motor9 -> Stationery : [Belt9==1]
  Motor7 -> Stationery : [Belt7==1]
  Stationery -> Motor7 [order 7] : [x==7&&y==7]
  Stationery -> Motor1 [order 1] : [x==1&&y==1]
  Motor1 -> Stationery : [Belt1==1]
  Stationery -> Motor2 [order 2] : [x==2&&y==2]
  Motor6 -> Stationery : [Belt6==1]
  Motor2 -> Stationery : [Belt2==1]
  Stationery -> Motor6 [order 6] : [x==6&&y==6]
  Motor5 -> Stationery : [Belt5==1]
  Stationery -> Motor5 [order 5] : [x==5&&y==5]
  (default) -> Stationery
  Motor4 -> Stationery : [Belt4==1]
  Stationery -> Motor4 [order 4] : [x==4&&y==4]
  Motor3 -> Stationery : [Belt3==1]
  Stationery -> Motor3 [order 3] : [x==3&&y==3]
  data: Belt1 input; Belt2 input; Belt3 input; Belt4 input; Belt5 input; Belt6 input; Belt7 input; Belt8 input; Belt9 input; x input; y input; V1 output; V2 output; V3 output; V4 output; V5 output; V6 output; V7 output; V8 output; V9 output
